simulink model "motor"  (R2023b)
settings: Solver=VariableStepAuto  StartTime=0.0  StopTime=40  RelTol=1e-3
values from neighbouring files (symbols this model uses):
  alpha = Rr/Lr    (= 3.74100719424)    [Lab7.m]
  beta = 1/gamma * Lm/(Ls*Lr)    (= 470.831419384)    [Lab7.m]
  fn = 50    [Lab7.m]
  gamma = 1 - Lm^2/(Ls*Lr)    (= 0.0492511651057)    [Lab7.m]
  J = 0.4    [Lab7.m]
  Kf = 0.1115    [Lab7.m]
  Lm = 0.041    [Lab7.m]
  Lr = 0.0417    [Lab7.m]
  Ls = 0.0424    [Lab7.m]
  Mr = 0    [Lab7.m]
  Rs = 0.294    [Lab7.m]
undefined symbols (not defined in the file or in its folder): denF, numF
settings Model: Creator=raluc  LastModifiedBy=raluc

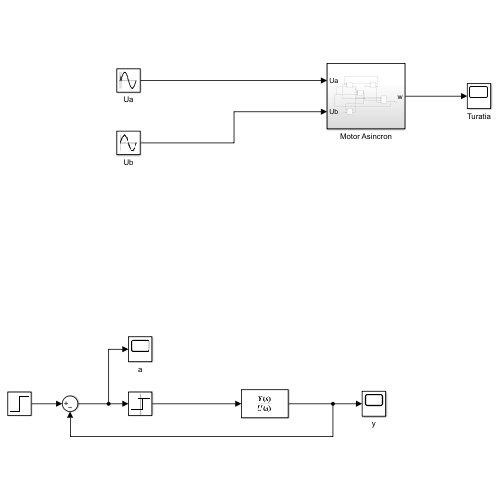
[thumbnail: Simulink's stored preview of the top-level diagram]
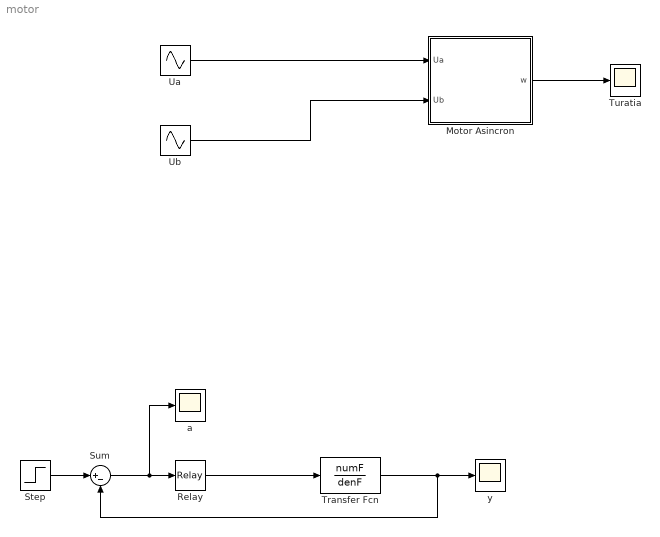
== system motor ==
  Motor Asincron : Subsystem
  Relay : Relay
  Step : Step  After=0  SampleTime=0
  Sum : Sum  Inputs=|+-
  Transfer Fcn : TransferFcn  Numerator=numF  Denominator=denF
  Turatia : Scope
  Ua : Sin  Amplitude=220*sqrt(2)  Frequency=2*pi*fn  Phase=pi/2  SampleTime=0
  Ub : Sin  Amplitude=220*sqrt(2)  Frequency=2*pi*fn  SampleTime=0
  a : Scope
  y : Scope
  wires:
  Motor Asincron/1(w) -> Turatia/1
  Ua/1 -> Motor Asincron/1(Ua)
  Ub/1 -> Motor Asincron/2(Ub)
  Relay/1 -> Transfer Fcn/1
  Sum/1 -> a/1, Relay/1
  Transfer Fcn/1 -> Sum/2, y/1
  Step/1 -> Sum/1

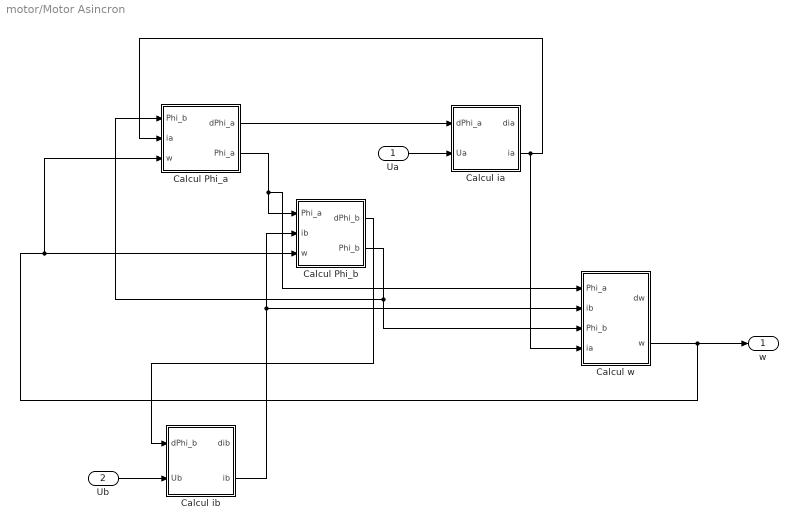
== system motor/Motor Asincron ==
  Ua : Inport
  Ub : Inport  Port=2
  Calcul Phi_a : Subsystem
  Calcul Phi_b : Subsystem
  Calcul ia : Subsystem
  Calcul ib : Subsystem
  Calcul w : Subsystem
  w : Outport
  wires:
  Calcul Phi_b/1(dPhi_b) -> Calcul ib/1(dPhi_b)
  Calcul ia/2(ia) -> Calcul w/4(ia), Calcul Phi_a/2(ia)
  Calcul ib/2(ib) -> Calcul w/2(ib), Calcul Phi_b/2(ib)
  Calcul Phi_a/2(Phi_a) -> Calcul w/1(Phi_a), Calcul Phi_b/1(Phi_a)
  Ua/1 -> Calcul ia/2(Ua)
  Calcul Phi_b/2(Phi_b) -> Calcul w/3(Phi_b), Calcul Phi_a/1(Phi_b)
  Ub/1 -> Calcul ib/2(Ub)
  Calcul Phi_a/1(dPhi_a) -> Calcul ia/1(dPhi_a)
  Calcul w/2(w) -> Calcul Phi_a/3(w), Calcul Phi_b/3(w), w/1

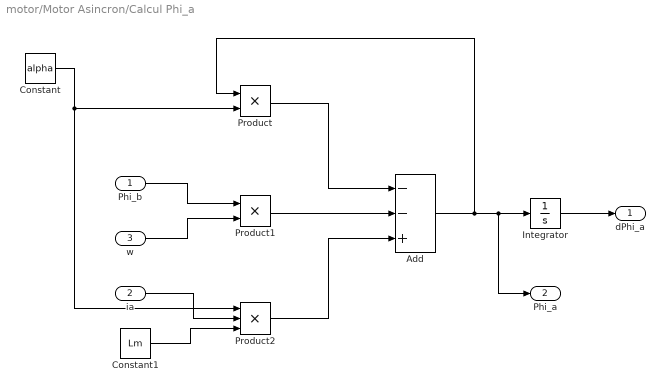
== system motor/Motor Asincron/Calcul Phi_a ==
  Phi_b : Inport
  ia : Inport  Port=2
  w : Inport  Port=3
  Add : Sum  Inputs=--+
  Constant : Constant  Value=alpha
  Constant1 : Constant  Value=Lm
  Integrator : Integrator
  Product : Product
  Product1 : Product
  Product2 : Product  Inputs=3
  dPhi_a : Outport
  Phi_a : Outport  Port=2
  wires:
  ia/1 -> Product2/2
  Constant1/1 -> Product2/3
  Product/1 -> Add/1
  Product2/1 -> Add/3
  Product1/1 -> Add/2
  Phi_b/1 -> Product1/1
  Add/1 -> Phi_a/1, Integrator/1, Product/1
  Constant/1 -> Product/2, Product2/1
  w/1 -> Product1/2
  Integrator/1 -> dPhi_a/1

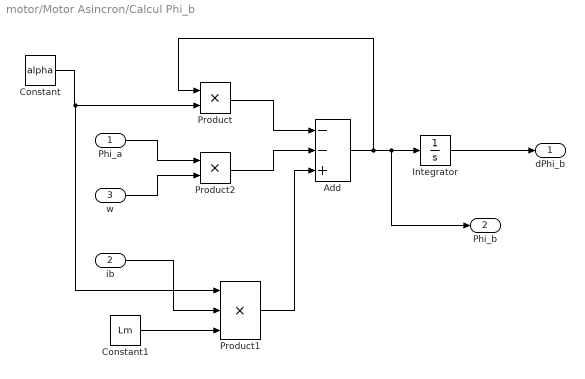
== system motor/Motor Asincron/Calcul Phi_b ==
  Phi_a : Inport
  ib : Inport  Port=2
  w : Inport  Port=3
  Add : Sum  Inputs=--+
  Constant : Constant  Value=alpha
  Constant1 : Constant  Value=Lm
  Integrator : Integrator
  Product : Product
  Product1 : Product  Inputs=3
  Product2 : Product
  dPhi_b : Outport
  Phi_b : Outport  Port=2
  wires:
  Constant/1 -> Product/2, Product1/1
  ib/1 -> Product1/2
  Product2/1 -> Add/2
  Product/1 -> Add/1
  w/1 -> Product2/2
  Phi_a/1 -> Product2/1
  Constant1/1 -> Product1/3
  Product1/1 -> Add/3
  Add/1 -> Phi_b/1, Integrator/1, Product/1
  Integrator/1 -> dPhi_b/1

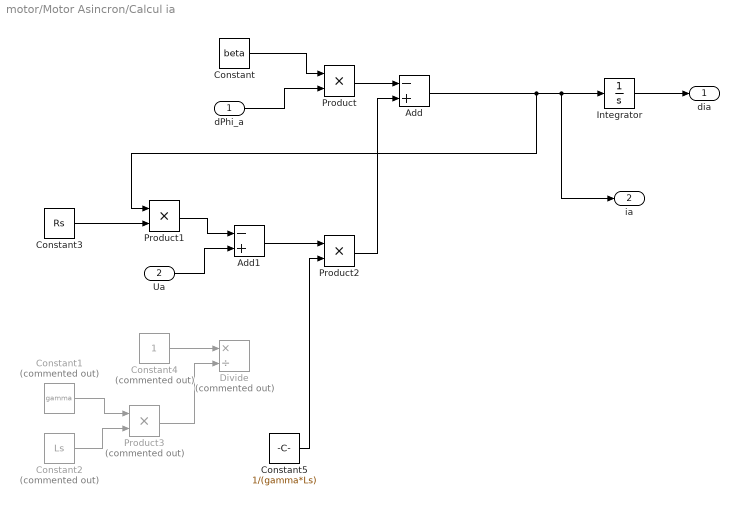
== system motor/Motor Asincron/Calcul ia ==
  dPhi_a : Inport
  Ua : Inport  Port=2
  Add : Sum  Inputs=-+
  Add1 : Sum  Inputs=-+
  Constant : Constant  Value=beta
  Constant1 : Constant  Commented=on  Value=gamma
  Constant2 : Constant  Commented=on  Value=Ls
  Constant3 : Constant  Value=Rs
  Constant4 : Constant  Commented=on
  Constant5 : Constant  Value=1/(gamma*Ls)
  Divide : Product  Commented=on  Inputs=*/
  Integrator : Integrator
  Product : Product
  Product1 : Product
  Product2 : Product
  Product3 : Product  Commented=on
  dia : Outport
  ia : Outport  Port=2
  wires:
  Add1/1 -> Product2/1
  Constant4/1 -> Divide/1
  Product2/1 -> Add/2
  dPhi_a/1 -> Product/2
  Constant/1 -> Product/1
  Add/1 -> ia/1, Integrator/1, Product1/1
  Constant2/1 -> Product3/2
  Product3/1 -> Divide/2
  Product/1 -> Add/1
  Ua/1 -> Add1/2
  Constant1/1 -> Product3/1
  Constant3/1 -> Product1/2
  Product1/1 -> Add1/1
  Integrator/1 -> dia/1
  Constant5/1 -> Product2/2

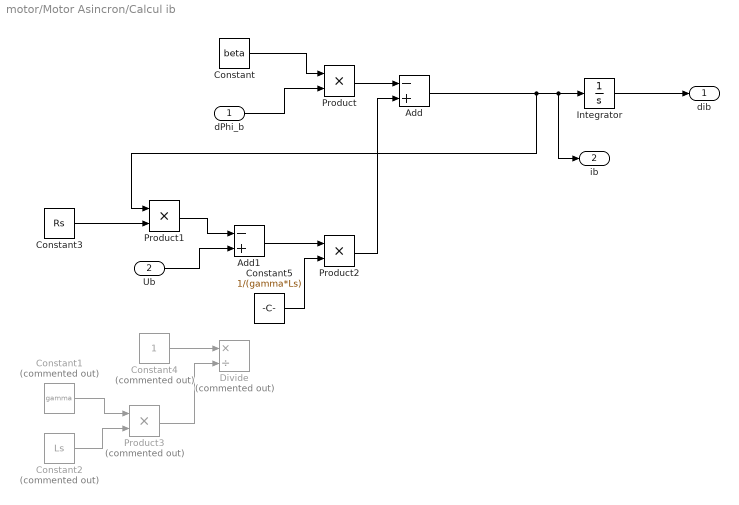
== system motor/Motor Asincron/Calcul ib ==
  dPhi_b : Inport
  Ub : Inport  Port=2
  Add : Sum  Inputs=-+
  Add1 : Sum  Inputs=-+
  Constant : Constant  Value=beta
  Constant1 : Constant  Commented=on  Value=gamma
  Constant2 : Constant  Commented=on  Value=Ls
  Constant3 : Constant  Value=Rs
  Constant4 : Constant  Commented=on
  Constant5 : Constant  Value=1/(gamma*Ls)
  Divide : Product  Commented=on  Inputs=*/
  Integrator : Integrator
  Product : Product
  Product1 : Product
  Product2 : Product
  Product3 : Product  Commented=on
  dib : Outport
  ib : Outport  Port=2
  wires:
  Constant1/1 -> Product3/1
  Add/1 -> Product1/1, ib/1, Integrator/1
  Constant/1 -> Product/1
  dPhi_b/1 -> Product/2
  Constant2/1 -> Product3/2
  Product2/1 -> Add/2
  Product/1 -> Add/1
  Add1/1 -> Product2/1
  Constant4/1 -> Divide/1
  Product1/1 -> Add1/1
  Product3/1 -> Divide/2
  Constant3/1 -> Product1/2
  Ub/1 -> Add1/2
  Integrator/1 -> dib/1
  Constant5/1 -> Product2/2

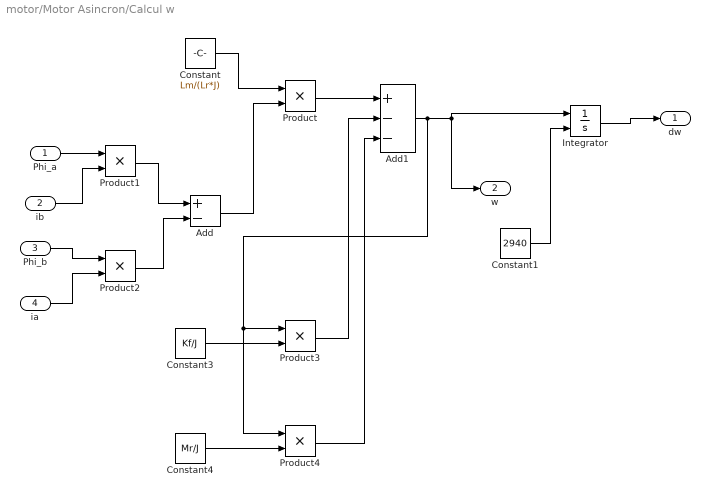
== system motor/Motor Asincron/Calcul w ==
  Phi_a : Inport
  ib : Inport  Port=2
  Phi_b : Inport  Port=3
  ia : Inport  Port=4
  Add : Sum  Inputs=+-
  Add1 : Sum  Inputs=+--
  Constant : Constant  Value=Lm/(Lr*J)
  Constant1 : Constant  Value=2940
  Constant3 : Constant  Value=Kf/J
  Constant4 : Constant  Value=Mr/J
  Integrator : Integrator  InitialConditionSource=external
  Product{,1..4} (5 alike) : Product
  dw : Outport
  w : Outport  Port=2
  wires:
  ib/1 -> Product1/2
  Constant3/1 -> Product3/2
  Add1/1 -> Product4/1, Product3/1, w/1, Integrator/1
  Product3/1 -> Add1/2
  ia/1 -> Product2/2
  Product1/1 -> Add/1
  Phi_a/1 -> Product1/1
  Product/1 -> Add1/1
  Product4/1 -> Add1/3
  Constant/1 -> Product/1
  Phi_b/1 -> Product2/1
  Product2/1 -> Add/2
  Add/1 -> Product/2
  Constant4/1 -> Product4/2
  Integrator/1 -> dw/1
  Constant1/1 -> Integrator/2
